simulink model "QuickStart"  (R2025a)
settings: Solver=VariableStepAuto  StartTime=0.0  StopTime=10.0  RelTol=1e-3
undefined symbols (not defined in the file): GND, GPIO, GPIO21, SCL, SDA
settings Model: Creator=el2jo  LastModifiedBy=el2jo

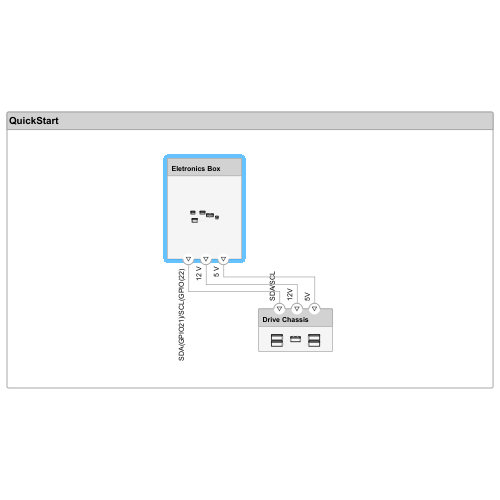
[thumbnail: Simulink's stored preview of the top-level diagram]
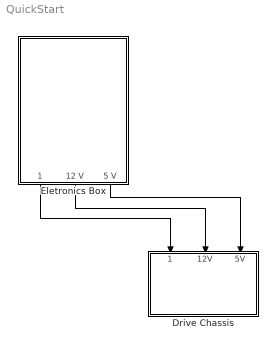
== system QuickStart ==
  Drive Chassis : Subsystem
      settings: PortSchema="{\"entries\":[{\"content\":{\"headerSize\":26,\"margin\":15,\"minimumSpacing\":25,\"sides\":[{\"content\":{},\"type\":\"ConnectorPlacement.EquallySpacedRectSide\",\"uuid\":\"48750758-9584-4908-8a58-a5fbbb9d9ec3\"},{\"content\":{\"side\":\"RIGHT\"},\"type\":\"ConnectorPlacement.EquallySpacedRectSide\",\"uuid\":\"52e2dad0-3097-421a-a882-362bd1258adc\"},{\"content\":{\"connectorIds\":[\"In1\",\"In2\",\"In3\"],\"side\":\"TOP\"},\"type\":\"ConnectorPlacement.EquallySpacedRectSide\",\"uuid\":\"e1803bf7-bd84-4e5d-8e9a-f8685f061664\"}]},\"type\":\"ConnectorPlacement.EquallySpacedConnector\",\"uuid\":\"5c436555-fc09-4a01-8a1e-11ce2b921fa0\"}],\"packageUris\":[\"http://schema.mathworks.com/mf0/Connector/R2020b\"],\"version\":\"1.0\"}"
  Eletronics Box : Subsystem
      settings: PortSchema="{\"entries\":[{\"content\":{\"headerSize\":26,\"margin\":15,\"minimumSpacing\":25,\"sides\":[{\"content\":{},\"type\":\"ConnectorPlacement.EquallySpacedRectSide\",\"uuid\":\"48750758-9584-4908-8a58-a5fbbb9d9ec3\"},{\"content\":{\"side\":\"RIGHT\"},\"type\":\"ConnectorPlacement.EquallySpacedRectSide\",\"uuid\":\"52e2dad0-3097-421a-a882-362bd1258adc\"},{\"content\":{\"side\":\"TOP\"},\"type\":\"ConnectorPlacement.EquallySpacedRectSide\",\"uuid\":\"e1803bf7-bd84-4e5d-8e9a-f8685f061664\"},{\"content\":{\"connectorIds\":[\"Out1\",\"Out2\",\"Out3\"],\"side\":\"BOTTOM\"},\"type\":\"ConnectorPlacement.EquallySpacedRectSide\",\"uuid\":\"9bfc03fe-8379-40b6-97ce-fe4ee1bc092f\"}]},\"type\":\"ConnectorPlacement.EquallySpacedConnector\",\"uuid\":\"5c436555-fc09-4a01-8a1e-11ce2b921fa0\"}],\"packageUris\":[\"http://schema.mathworks.com/mf0/Connector/R2020b\"],\"version\":\"1.0\"}"
  wires:
  Eletronics Box/3(5 V) -> Drive Chassis/3(5V)
  Eletronics Box/1("SDA(GPIO21)/SCL(GPIO(22) ") -> Drive Chassis/1(SDA/SCL)
  Eletronics Box/2(12 V) -> Drive Chassis/2(12V)

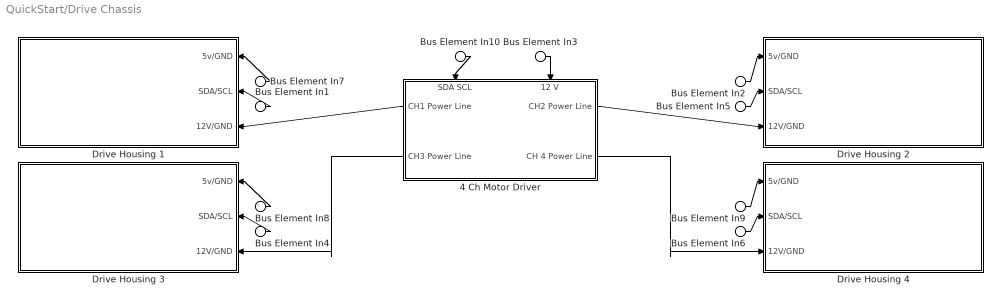
== system QuickStart/Drive Chassis ==
  Bus Element In{1,4..6,10} (5 alike) : Inport  PortName=SDA/SCL
  Bus Element In3 : Inport  Port=2  PortName=12V
  Bus Element In{2,7..9} (4 alike) : Inport  Port=3  PortName=5V
  4 Ch Motor Driver : Subsystem
      settings: PortSchema="{\"entries\":[{\"content\":{\"headerSize\":26,\"margin\":15,\"minimumSpacing\":25,\"sides\":[{\"content\":{\"connectorIds\":[\"Out1\",\"Out3\"]},\"type\":\"ConnectorPlacement.EquallySpacedRectSide\",\"uuid\":\"48750758-9584-4908-8a58-a5fbbb9d9ec3\"},{\"content\":{\"connectorIds\":[\"Out2\",\"Out4\"],\"side\":\"RIGHT\"},\"type\":\"ConnectorPlacement.EquallySpacedRectSide\",\"uuid\":\"52e2dad0-3097-421a-a882-362bd1258adc\"},{\"content\":{\"connectorIds\":[\"In1\",\"In2\"],\"side\":\"TOP\"},\"type\":\"ConnectorPlacement.EquallySpacedRectSide\",\"uuid\":\"e1803bf7-bd84-4e5d-8e9a-f8685f061664\"}]},\"type\":\"ConnectorPlacement.EquallySpacedConnector\",\"uuid\":\"5c436555-fc09-4a01-8a1e-11ce2b921fa0\"}],\"packageUris\":[\"http://schema.mathworks.com/mf0/Connector/R2020b\"],\"version\":\"1.0\"}"
  Drive Housing 1 : Subsystem
      settings: PortSchema="{\"entries\":[{\"content\":{\"headerSize\":26,\"margin\":15,\"minimumSpacing\":25,\"sides\":[{\"content\":{},\"type\":\"ConnectorPlacement.EquallySpacedRectSide\",\"uuid\":\"e7607396-8c96-4a6c-8f29-b5a2e3597902\"},{\"content\":{\"connectorIds\":[\"In1\",\"In2\",\"In3\"],\"side\":\"RIGHT\"},\"type\":\"ConnectorPlacement.EquallySpacedRectSide\",\"uuid\":\"459ece88-82a0-4a1d-ada4-6a68a35fe0a8\"},{\"content\":{\"side\":\"TOP\"},\"type\":\"ConnectorPlacement.EquallySpacedRectSide\",\"uuid\":\"796374a7-05ea-42d9-8bb3-fc90485df8c0\"}]},\"type\":\"ConnectorPlacement.EquallySpacedConnector\",\"uuid\":\"d0e626ee-7e22-4847-893e-8ab9090f2344\"}],\"packageUris\":[\"http://schema.mathworks.com/mf0/Connector/R2020b\"],\"version\":\"1.0\"}"
  Drive Housing 2 : Subsystem
      settings: PortSchema="{\"entries\":[{\"content\":{\"headerSize\":26,\"margin\":15,\"minimumSpacing\":25,\"sides\":[{\"content\":{\"connectorIds\":[\"In1\",\"In2\",\"In3\"]},\"type\":\"ConnectorPlacement.EquallySpacedRectSide\",\"uuid\":\"e7607396-8c96-4a6c-8f29-b5a2e3597902\"},{\"content\":{\"side\":\"RIGHT\"},\"type\":\"ConnectorPlacement.EquallySpacedRectSide\",\"uuid\":\"459ece88-82a0-4a1d-ada4-6a68a35fe0a8\"},{\"content\":{\"side\":\"TOP\"},\"type\":\"ConnectorPlacement.EquallySpacedRectSide\",\"uuid\":\"796374a7-05ea-42d9-8bb3-fc90485df8c0\"}]},\"type\":\"ConnectorPlacement.EquallySpacedConnector\",\"uuid\":\"d0e626ee-7e22-4847-893e-8ab9090f2344\"}],\"packageUris\":[\"http://schema.mathworks.com/mf0/Connector/R2020b\"],\"version\":\"1.0\"}"
  Drive Housing 3 : Subsystem
      settings: PortSchema="{\"entries\":[{\"content\":{\"headerSize\":26,\"margin\":15,\"minimumSpacing\":25,\"sides\":[{\"content\":{},\"type\":\"ConnectorPlacement.EquallySpacedRectSide\",\"uuid\":\"e7607396-8c96-4a6c-8f29-b5a2e3597902\"},{\"content\":{\"connectorIds\":[\"In1\",\"In2\",\"In3\"],\"side\":\"RIGHT\"},\"type\":\"ConnectorPlacement.EquallySpacedRectSide\",\"uuid\":\"459ece88-82a0-4a1d-ada4-6a68a35fe0a8\"},{\"content\":{\"side\":\"TOP\"},\"type\":\"ConnectorPlacement.EquallySpacedRectSide\",\"uuid\":\"796374a7-05ea-42d9-8bb3-fc90485df8c0\"}]},\"type\":\"ConnectorPlacement.EquallySpacedConnector\",\"uuid\":\"d0e626ee-7e22-4847-893e-8ab9090f2344\"}],\"packageUris\":[\"http://schema.mathworks.com/mf0/Connector/R2020b\"],\"version\":\"1.0\"}"
  Drive Housing 4 : Subsystem
      settings: PortSchema="{\"entries\":[{\"content\":{\"headerSize\":26,\"margin\":15,\"minimumSpacing\":25,\"sides\":[{\"content\":{\"connectorIds\":[\"In1\",\"In2\",\"In3\"]},\"type\":\"ConnectorPlacement.EquallySpacedRectSide\",\"uuid\":\"e7607396-8c96-4a6c-8f29-b5a2e3597902\"},{\"content\":{\"side\":\"RIGHT\"},\"type\":\"ConnectorPlacement.EquallySpacedRectSide\",\"uuid\":\"459ece88-82a0-4a1d-ada4-6a68a35fe0a8\"},{\"content\":{\"side\":\"TOP\"},\"type\":\"ConnectorPlacement.EquallySpacedRectSide\",\"uuid\":\"796374a7-05ea-42d9-8bb3-fc90485df8c0\"}]},\"type\":\"ConnectorPlacement.EquallySpacedConnector\",\"uuid\":\"d0e626ee-7e22-4847-893e-8ab9090f2344\"}],\"packageUris\":[\"http://schema.mathworks.com/mf0/Connector/R2020b\"],\"version\":\"1.0\"}"
  wires:
  4 Ch Motor Driver/4(CH 4 Power Line) -> Drive Housing 4/3(12V/GND)
  4 Ch Motor Driver/2(CH2 Power Line) -> Drive Housing 2/3(12V/GND)
  4 Ch Motor Driver/3(CH3 Power Line) -> Drive Housing 3/3(12V/GND)
  4 Ch Motor Driver/1(CH1 Power Line) -> Drive Housing 1/3(12V/GND)
  Bus Element In1/1 -> Drive Housing 1/2(SDA/SCL)
  Bus Element In4/1 -> Drive Housing 3/2(SDA/SCL)
  Bus Element In5/1 -> Drive Housing 2/2(SDA/SCL)
  Bus Element In6/1 -> Drive Housing 4/2(SDA/SCL)
  Bus Element In2/1 -> Drive Housing 2/1(5v/GND)
  Bus Element In7/1 -> Drive Housing 1/1(5v/GND)
  Bus Element In8/1 -> Drive Housing 3/1(5v/GND)
  Bus Element In9/1 -> Drive Housing 4/1(5v/GND)
  Bus Element In10/1 -> 4 Ch Motor Driver/1(SDA SCL)
  Bus Element In3/1 -> 4 Ch Motor Driver/2("12 V ")

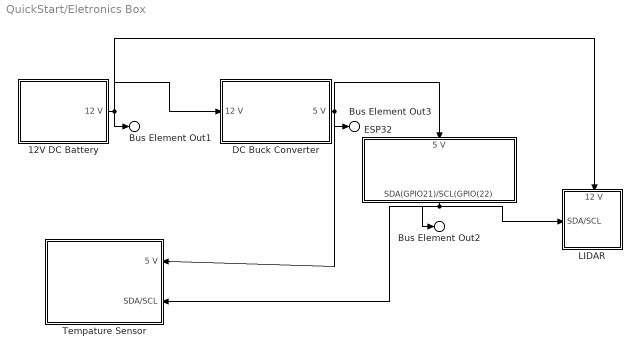
== system QuickStart/Eletronics Box ==
  12V DC Battery : Subsystem
      settings: PortSchema="{\"entries\":[{\"content\":{\"headerSize\":26,\"margin\":15,\"minimumSpacing\":25,\"sides\":[{\"content\":{},\"type\":\"ConnectorPlacement.EquallySpacedRectSide\",\"uuid\":\"48750758-9584-4908-8a58-a5fbbb9d9ec3\"},{\"content\":{\"connectorIds\":[\"Out1\"],\"side\":\"RIGHT\"},\"type\":\"ConnectorPlacement.EquallySpacedRectSide\",\"uuid\":\"52e2dad0-3097-421a-a882-362bd1258adc\"},{\"content\":{\"side\":\"TOP\"},\"type\":\"ConnectorPlacement.EquallySpacedRectSide\",\"uuid\":\"e1803bf7-bd84-4e5d-8e9a-f8685f061664\"}]},\"type\":\"ConnectorPlacement.EquallySpacedConnector\",\"uuid\":\"5c436555-fc09-4a01-8a1e-11ce2b921fa0\"}],\"packageUris\":[\"http://schema.mathworks.com/mf0/Connector/R2020b\"],\"version\":\"1.0\"}"
  DC Buck Converter : Subsystem
      settings: PortSchema="{\"entries\":[{\"content\":{\"headerSize\":26,\"margin\":15,\"minimumSpacing\":25,\"sides\":[{\"content\":{\"connectorIds\":[\"In1\"]},\"type\":\"ConnectorPlacement.EquallySpacedRectSide\",\"uuid\":\"48750758-9584-4908-8a58-a5fbbb9d9ec3\"},{\"content\":{\"connectorIds\":[\"Out1\"],\"side\":\"RIGHT\"},\"type\":\"ConnectorPlacement.EquallySpacedRectSide\",\"uuid\":\"52e2dad0-3097-421a-a882-362bd1258adc\"},{\"content\":{\"side\":\"TOP\"},\"type\":\"ConnectorPlacement.EquallySpacedRectSide\",\"uuid\":\"e1803bf7-bd84-4e5d-8e9a-f8685f061664\"}]},\"type\":\"ConnectorPlacement.EquallySpacedConnector\",\"uuid\":\"5c436555-fc09-4a01-8a1e-11ce2b921fa0\"}],\"packageUris\":[\"http://schema.mathworks.com/mf0/Connector/R2020b\"],\"version\":\"1.0\"}"
  ESP32 : Subsystem
      settings: PortSchema="{\"entries\":[{\"content\":{\"headerSize\":26,\"margin\":15,\"minimumSpacing\":25,\"sides\":[{\"content\":{},\"type\":\"ConnectorPlacement.EquallySpacedRectSide\",\"uuid\":\"48750758-9584-4908-8a58-a5fbbb9d9ec3\"},{\"content\":{\"side\":\"RIGHT\"},\"type\":\"ConnectorPlacement.EquallySpacedRectSide\",\"uuid\":\"52e2dad0-3097-421a-a882-362bd1258adc\"},{\"content\":{\"connectorIds\":[\"In1\"],\"side\":\"TOP\"},\"type\":\"ConnectorPlacement.EquallySpacedRectSide\",\"uuid\":\"e1803bf7-bd84-4e5d-8e9a-f8685f061664\"},{\"content\":{\"connectorIds\":[\"Out1\"],\"side\":\"BOTTOM\"},\"type\":\"ConnectorPlacement.EquallySpacedRectSide\",\"uuid\":\"3c1c43d4-aa76-4122-9080-ecb1da993d45\"}]},\"type\":\"ConnectorPlacement.EquallySpacedConnector\",\"uuid\":\"5c436555-fc09-4a01-8a1e-11ce2b921fa0\"}],\"packageUris\":[\"http://schema.mathworks.com/mf0/Connector/R2020b\"],\"version\":\"1.0\"}"
  LIDAR : Subsystem
      settings: PortSchema="{\"entries\":[{\"content\":{\"headerSize\":26,\"margin\":15,\"minimumSpacing\":25,\"sides\":[{\"content\":{\"connectorIds\":[\"In1\"]},\"type\":\"ConnectorPlacement.EquallySpacedRectSide\",\"uuid\":\"48750758-9584-4908-8a58-a5fbbb9d9ec3\"},{\"content\":{\"side\":\"RIGHT\"},\"type\":\"ConnectorPlacement.EquallySpacedRectSide\",\"uuid\":\"52e2dad0-3097-421a-a882-362bd1258adc\"},{\"content\":{\"connectorIds\":[\"In2\"],\"side\":\"TOP\"},\"type\":\"ConnectorPlacement.EquallySpacedRectSide\",\"uuid\":\"e1803bf7-bd84-4e5d-8e9a-f8685f061664\"}]},\"type\":\"ConnectorPlacement.EquallySpacedConnector\",\"uuid\":\"5c436555-fc09-4a01-8a1e-11ce2b921fa0\"}],\"packageUris\":[\"http://schema.mathworks.com/mf0/Connector/R2020b\"],\"version\":\"1.0\"}"
  Tempature Sensor : Subsystem
      settings: PortSchema="{\"entries\":[{\"content\":{\"headerSize\":26,\"margin\":15,\"minimumSpacing\":25,\"sides\":[{\"content\":{},\"type\":\"ConnectorPlacement.EquallySpacedRectSide\",\"uuid\":\"48750758-9584-4908-8a58-a5fbbb9d9ec3\"},{\"content\":{\"connectorIds\":[\"In1\",\"In2\"],\"side\":\"RIGHT\"},\"type\":\"ConnectorPlacement.EquallySpacedRectSide\",\"uuid\":\"52e2dad0-3097-421a-a882-362bd1258adc\"},{\"content\":{\"side\":\"TOP\"},\"type\":\"ConnectorPlacement.EquallySpacedRectSide\",\"uuid\":\"e1803bf7-bd84-4e5d-8e9a-f8685f061664\"}]},\"type\":\"ConnectorPlacement.EquallySpacedConnector\",\"uuid\":\"5c436555-fc09-4a01-8a1e-11ce2b921fa0\"}],\"packageUris\":[\"http://schema.mathworks.com/mf0/Connector/R2020b\"],\"version\":\"1.0\"}"
  Bus Element Out2 : Outport  PortName=SDA(GPIO21)/SCL(GPIO(22)
  Bus Element Out1 : Outport  Port=2  PortName=12 V
  Bus Element Out3 : Outport  Port=3  PortName=5 V
  wires:
  12V DC Battery/1(12 V) -> Bus Element Out1/1, DC Buck Converter/1(12 V), LIDAR/2(12 V)
  ESP32/1("SDA(GPIO21)/SCL(GPIO(22) ") -> Bus Element Out2/1, Tempature Sensor/2(SDA/SCL), LIDAR/1(SDA/SCL)
  DC Buck Converter/1(5 V) -> Bus Element Out3/1, Tempature Sensor/1(5 V), ESP32/1(5 V)

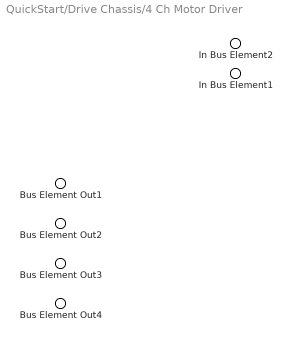
== system QuickStart/Drive Chassis/4 Ch Motor Driver ==
  In Bus Element1 : Inport  PortName=SDA SCL
  In Bus Element2 : Inport  Port=2  PortName=12 V
  Bus Element Out1 : Outport  PortName=CH1 Power Line
  Bus Element Out2 : Outport  Port=2  PortName=CH2 Power Line
  Bus Element Out3 : Outport  Port=3  PortName=CH3 Power Line
  Bus Element Out4 : Outport  Port=4  PortName=CH 4 Power Line

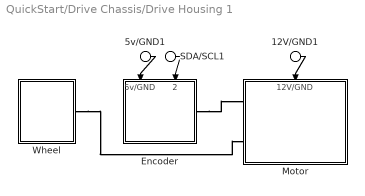
== system QuickStart/Drive Chassis/Drive Housing 1 ==
  5v/GND1 : Inport  PortName=5v/GND
  SDA/SCL1 : Inport  Port=2  PortName=SDA/SCL
  12V/GND1 : Inport  Port=3  PortName=12V/GND
  "Encoder " : Subsystem
      settings: PortSchema="{\"entries\":[{\"content\":{\"headerSize\":26,\"margin\":15,\"minimumSpacing\":25,\"sides\":[{\"content\":{},\"type\":\"ConnectorPlacement.EquallySpacedRectSide\",\"uuid\":\"48750758-9584-4908-8a58-a5fbbb9d9ec3\"},{\"content\":{\"connectorIds\":[\"RConn1\"],\"side\":\"RIGHT\"},\"type\":\"ConnectorPlacement.EquallySpacedRectSide\",\"uuid\":\"52e2dad0-3097-421a-a882-362bd1258adc\"},{\"content\":{\"connectorIds\":[\"In1\",\"In2\"],\"side\":\"TOP\"},\"type\":\"ConnectorPlacement.EquallySpacedRectSide\",\"uuid\":\"e1803bf7-bd84-4e5d-8e9a-f8685f061664\"}]},\"type\":\"ConnectorPlacement.EquallySpacedConnector\",\"uuid\":\"5c436555-fc09-4a01-8a1e-11ce2b921fa0\"}],\"packageUris\":[\"http://schema.mathworks.com/mf0/Connector/R2020b\"],\"version\":\"1.0\"}"
  Motor : Subsystem
      settings: PortSchema="{\"entries\":[{\"content\":{\"headerSize\":26,\"margin\":15,\"minimumSpacing\":25,\"sides\":[{\"content\":{\"connectorIds\":[\"LConn1\",\"LConn2\"]},\"type\":\"ConnectorPlacement.EquallySpacedRectSide\",\"uuid\":\"48750758-9584-4908-8a58-a5fbbb9d9ec3\"},{\"content\":{\"side\":\"RIGHT\"},\"type\":\"ConnectorPlacement.EquallySpacedRectSide\",\"uuid\":\"52e2dad0-3097-421a-a882-362bd1258adc\"},{\"content\":{\"connectorIds\":[\"In1\"],\"side\":\"TOP\"},\"type\":\"ConnectorPlacement.EquallySpacedRectSide\",\"uuid\":\"e1803bf7-bd84-4e5d-8e9a-f8685f061664\"}]},\"type\":\"ConnectorPlacement.EquallySpacedConnector\",\"uuid\":\"5c436555-fc09-4a01-8a1e-11ce2b921fa0\"}],\"packageUris\":[\"http://schema.mathworks.com/mf0/Connector/R2020b\"],\"version\":\"1.0\"}"
  Wheel : Subsystem
      settings: PortSchema="{\"entries\":[{\"content\":{\"headerSize\":26,\"margin\":15,\"minimumSpacing\":25,\"sides\":[{\"content\":{},\"type\":\"ConnectorPlacement.EquallySpacedRectSide\",\"uuid\":\"48750758-9584-4908-8a58-a5fbbb9d9ec3\"},{\"content\":{\"connectorIds\":[\"RConn1\"],\"side\":\"RIGHT\"},\"type\":\"ConnectorPlacement.EquallySpacedRectSide\",\"uuid\":\"52e2dad0-3097-421a-a882-362bd1258adc\"},{\"content\":{\"side\":\"TOP\"},\"type\":\"ConnectorPlacement.EquallySpacedRectSide\",\"uuid\":\"e1803bf7-bd84-4e5d-8e9a-f8685f061664\"}]},\"type\":\"ConnectorPlacement.EquallySpacedConnector\",\"uuid\":\"5c436555-fc09-4a01-8a1e-11ce2b921fa0\"}],\"packageUris\":[\"http://schema.mathworks.com/mf0/Connector/R2020b\"],\"version\":\"1.0\"}"
  wires:
  5v/GND1/1 -> "Encoder "/1(5v/GND)
  SDA/SCL1/1 -> "Encoder "/2(SDA/SCL)
  12V/GND1/1 -> Motor/1(12V/GND)
  connections:
  "Encoder "/RConn1 -- Motor/LConn1
  Wheel/RConn1 -- Motor/LConn2

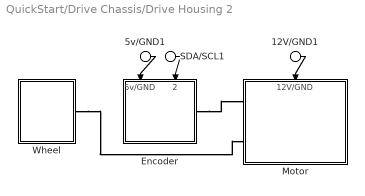
== system QuickStart/Drive Chassis/Drive Housing 2 ==
  5v/GND1 : Inport  PortName=5v/GND
  SDA/SCL1 : Inport  Port=2  PortName=SDA/SCL
  12V/GND1 : Inport  Port=3  PortName=12V/GND
  "Encoder " : Subsystem
      settings: PortSchema="{\"entries\":[{\"content\":{\"headerSize\":26,\"margin\":15,\"minimumSpacing\":25,\"sides\":[{\"content\":{},\"type\":\"ConnectorPlacement.EquallySpacedRectSide\",\"uuid\":\"48750758-9584-4908-8a58-a5fbbb9d9ec3\"},{\"content\":{\"connectorIds\":[\"RConn1\"],\"side\":\"RIGHT\"},\"type\":\"ConnectorPlacement.EquallySpacedRectSide\",\"uuid\":\"52e2dad0-3097-421a-a882-362bd1258adc\"},{\"content\":{\"connectorIds\":[\"In1\",\"In2\"],\"side\":\"TOP\"},\"type\":\"ConnectorPlacement.EquallySpacedRectSide\",\"uuid\":\"e1803bf7-bd84-4e5d-8e9a-f8685f061664\"}]},\"type\":\"ConnectorPlacement.EquallySpacedConnector\",\"uuid\":\"5c436555-fc09-4a01-8a1e-11ce2b921fa0\"}],\"packageUris\":[\"http://schema.mathworks.com/mf0/Connector/R2020b\"],\"version\":\"1.0\"}"
  Motor : Subsystem
      settings: PortSchema="{\"entries\":[{\"content\":{\"headerSize\":26,\"margin\":15,\"minimumSpacing\":25,\"sides\":[{\"content\":{\"connectorIds\":[\"LConn1\",\"LConn2\"]},\"type\":\"ConnectorPlacement.EquallySpacedRectSide\",\"uuid\":\"48750758-9584-4908-8a58-a5fbbb9d9ec3\"},{\"content\":{\"side\":\"RIGHT\"},\"type\":\"ConnectorPlacement.EquallySpacedRectSide\",\"uuid\":\"52e2dad0-3097-421a-a882-362bd1258adc\"},{\"content\":{\"connectorIds\":[\"In1\"],\"side\":\"TOP\"},\"type\":\"ConnectorPlacement.EquallySpacedRectSide\",\"uuid\":\"e1803bf7-bd84-4e5d-8e9a-f8685f061664\"}]},\"type\":\"ConnectorPlacement.EquallySpacedConnector\",\"uuid\":\"5c436555-fc09-4a01-8a1e-11ce2b921fa0\"}],\"packageUris\":[\"http://schema.mathworks.com/mf0/Connector/R2020b\"],\"version\":\"1.0\"}"
  Wheel : Subsystem
      settings: PortSchema="{\"entries\":[{\"content\":{\"headerSize\":26,\"margin\":15,\"minimumSpacing\":25,\"sides\":[{\"content\":{},\"type\":\"ConnectorPlacement.EquallySpacedRectSide\",\"uuid\":\"48750758-9584-4908-8a58-a5fbbb9d9ec3\"},{\"content\":{\"connectorIds\":[\"RConn1\"],\"side\":\"RIGHT\"},\"type\":\"ConnectorPlacement.EquallySpacedRectSide\",\"uuid\":\"52e2dad0-3097-421a-a882-362bd1258adc\"},{\"content\":{\"side\":\"TOP\"},\"type\":\"ConnectorPlacement.EquallySpacedRectSide\",\"uuid\":\"e1803bf7-bd84-4e5d-8e9a-f8685f061664\"}]},\"type\":\"ConnectorPlacement.EquallySpacedConnector\",\"uuid\":\"5c436555-fc09-4a01-8a1e-11ce2b921fa0\"}],\"packageUris\":[\"http://schema.mathworks.com/mf0/Connector/R2020b\"],\"version\":\"1.0\"}"
  wires:
  5v/GND1/1 -> "Encoder "/1(5v/GND)
  SDA/SCL1/1 -> "Encoder "/2(SDA/SCL)
  12V/GND1/1 -> Motor/1(12V/GND)
  connections:
  "Encoder "/RConn1 -- Motor/LConn1
  Wheel/RConn1 -- Motor/LConn2

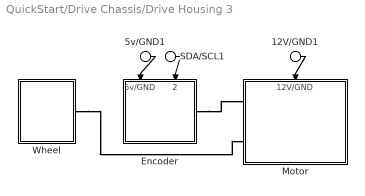
== system QuickStart/Drive Chassis/Drive Housing 3 ==
  5v/GND1 : Inport  PortName=5v/GND
  SDA/SCL1 : Inport  Port=2  PortName=SDA/SCL
  12V/GND1 : Inport  Port=3  PortName=12V/GND
  "Encoder " : Subsystem
      settings: PortSchema="{\"entries\":[{\"content\":{\"headerSize\":26,\"margin\":15,\"minimumSpacing\":25,\"sides\":[{\"content\":{},\"type\":\"ConnectorPlacement.EquallySpacedRectSide\",\"uuid\":\"48750758-9584-4908-8a58-a5fbbb9d9ec3\"},{\"content\":{\"connectorIds\":[\"RConn1\"],\"side\":\"RIGHT\"},\"type\":\"ConnectorPlacement.EquallySpacedRectSide\",\"uuid\":\"52e2dad0-3097-421a-a882-362bd1258adc\"},{\"content\":{\"connectorIds\":[\"In1\",\"In2\"],\"side\":\"TOP\"},\"type\":\"ConnectorPlacement.EquallySpacedRectSide\",\"uuid\":\"e1803bf7-bd84-4e5d-8e9a-f8685f061664\"}]},\"type\":\"ConnectorPlacement.EquallySpacedConnector\",\"uuid\":\"5c436555-fc09-4a01-8a1e-11ce2b921fa0\"}],\"packageUris\":[\"http://schema.mathworks.com/mf0/Connector/R2020b\"],\"version\":\"1.0\"}"
  Motor : Subsystem
      settings: PortSchema="{\"entries\":[{\"content\":{\"headerSize\":26,\"margin\":15,\"minimumSpacing\":25,\"sides\":[{\"content\":{\"connectorIds\":[\"LConn1\",\"LConn2\"]},\"type\":\"ConnectorPlacement.EquallySpacedRectSide\",\"uuid\":\"48750758-9584-4908-8a58-a5fbbb9d9ec3\"},{\"content\":{\"side\":\"RIGHT\"},\"type\":\"ConnectorPlacement.EquallySpacedRectSide\",\"uuid\":\"52e2dad0-3097-421a-a882-362bd1258adc\"},{\"content\":{\"connectorIds\":[\"In1\"],\"side\":\"TOP\"},\"type\":\"ConnectorPlacement.EquallySpacedRectSide\",\"uuid\":\"e1803bf7-bd84-4e5d-8e9a-f8685f061664\"}]},\"type\":\"ConnectorPlacement.EquallySpacedConnector\",\"uuid\":\"5c436555-fc09-4a01-8a1e-11ce2b921fa0\"}],\"packageUris\":[\"http://schema.mathworks.com/mf0/Connector/R2020b\"],\"version\":\"1.0\"}"
  Wheel : Subsystem
      settings: PortSchema="{\"entries\":[{\"content\":{\"headerSize\":26,\"margin\":15,\"minimumSpacing\":25,\"sides\":[{\"content\":{},\"type\":\"ConnectorPlacement.EquallySpacedRectSide\",\"uuid\":\"48750758-9584-4908-8a58-a5fbbb9d9ec3\"},{\"content\":{\"connectorIds\":[\"RConn1\"],\"side\":\"RIGHT\"},\"type\":\"ConnectorPlacement.EquallySpacedRectSide\",\"uuid\":\"52e2dad0-3097-421a-a882-362bd1258adc\"},{\"content\":{\"side\":\"TOP\"},\"type\":\"ConnectorPlacement.EquallySpacedRectSide\",\"uuid\":\"e1803bf7-bd84-4e5d-8e9a-f8685f061664\"}]},\"type\":\"ConnectorPlacement.EquallySpacedConnector\",\"uuid\":\"5c436555-fc09-4a01-8a1e-11ce2b921fa0\"}],\"packageUris\":[\"http://schema.mathworks.com/mf0/Connector/R2020b\"],\"version\":\"1.0\"}"
  wires:
  5v/GND1/1 -> "Encoder "/1(5v/GND)
  SDA/SCL1/1 -> "Encoder "/2(SDA/SCL)
  12V/GND1/1 -> Motor/1(12V/GND)
  connections:
  "Encoder "/RConn1 -- Motor/LConn1
  Wheel/RConn1 -- Motor/LConn2

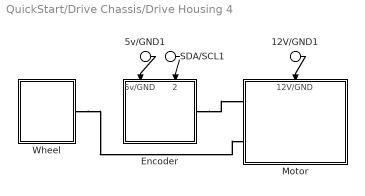
== system QuickStart/Drive Chassis/Drive Housing 4 ==
  5v/GND1 : Inport  PortName=5v/GND
  SDA/SCL1 : Inport  Port=2  PortName=SDA/SCL
  12V/GND1 : Inport  Port=3  PortName=12V/GND
  "Encoder " : Subsystem
      settings: PortSchema="{\"entries\":[{\"content\":{\"headerSize\":26,\"margin\":15,\"minimumSpacing\":25,\"sides\":[{\"content\":{},\"type\":\"ConnectorPlacement.EquallySpacedRectSide\",\"uuid\":\"48750758-9584-4908-8a58-a5fbbb9d9ec3\"},{\"content\":{\"connectorIds\":[\"RConn1\"],\"side\":\"RIGHT\"},\"type\":\"ConnectorPlacement.EquallySpacedRectSide\",\"uuid\":\"52e2dad0-3097-421a-a882-362bd1258adc\"},{\"content\":{\"connectorIds\":[\"In1\",\"In2\"],\"side\":\"TOP\"},\"type\":\"ConnectorPlacement.EquallySpacedRectSide\",\"uuid\":\"e1803bf7-bd84-4e5d-8e9a-f8685f061664\"}]},\"type\":\"ConnectorPlacement.EquallySpacedConnector\",\"uuid\":\"5c436555-fc09-4a01-8a1e-11ce2b921fa0\"}],\"packageUris\":[\"http://schema.mathworks.com/mf0/Connector/R2020b\"],\"version\":\"1.0\"}"
  Motor : Subsystem
      settings: PortSchema="{\"entries\":[{\"content\":{\"headerSize\":26,\"margin\":15,\"minimumSpacing\":25,\"sides\":[{\"content\":{\"connectorIds\":[\"LConn1\",\"LConn2\"]},\"type\":\"ConnectorPlacement.EquallySpacedRectSide\",\"uuid\":\"48750758-9584-4908-8a58-a5fbbb9d9ec3\"},{\"content\":{\"side\":\"RIGHT\"},\"type\":\"ConnectorPlacement.EquallySpacedRectSide\",\"uuid\":\"52e2dad0-3097-421a-a882-362bd1258adc\"},{\"content\":{\"connectorIds\":[\"In1\"],\"side\":\"TOP\"},\"type\":\"ConnectorPlacement.EquallySpacedRectSide\",\"uuid\":\"e1803bf7-bd84-4e5d-8e9a-f8685f061664\"}]},\"type\":\"ConnectorPlacement.EquallySpacedConnector\",\"uuid\":\"5c436555-fc09-4a01-8a1e-11ce2b921fa0\"}],\"packageUris\":[\"http://schema.mathworks.com/mf0/Connector/R2020b\"],\"version\":\"1.0\"}"
  Wheel : Subsystem
      settings: PortSchema="{\"entries\":[{\"content\":{\"headerSize\":26,\"margin\":15,\"minimumSpacing\":25,\"sides\":[{\"content\":{},\"type\":\"ConnectorPlacement.EquallySpacedRectSide\",\"uuid\":\"48750758-9584-4908-8a58-a5fbbb9d9ec3\"},{\"content\":{\"connectorIds\":[\"RConn1\"],\"side\":\"RIGHT\"},\"type\":\"ConnectorPlacement.EquallySpacedRectSide\",\"uuid\":\"52e2dad0-3097-421a-a882-362bd1258adc\"},{\"content\":{\"side\":\"TOP\"},\"type\":\"ConnectorPlacement.EquallySpacedRectSide\",\"uuid\":\"e1803bf7-bd84-4e5d-8e9a-f8685f061664\"}]},\"type\":\"ConnectorPlacement.EquallySpacedConnector\",\"uuid\":\"5c436555-fc09-4a01-8a1e-11ce2b921fa0\"}],\"packageUris\":[\"http://schema.mathworks.com/mf0/Connector/R2020b\"],\"version\":\"1.0\"}"
  wires:
  5v/GND1/1 -> "Encoder "/1(5v/GND)
  SDA/SCL1/1 -> "Encoder "/2(SDA/SCL)
  12V/GND1/1 -> Motor/1(12V/GND)
  connections:
  "Encoder "/RConn1 -- Motor/LConn1
  Wheel/RConn1 -- Motor/LConn2

== system QuickStart/Eletronics Box/12V DC Battery ==
  Bus Element Out1 : Outport  PortName=12 V

== system QuickStart/Eletronics Box/DC Buck Converter ==
  Bus Element In1 : Inport  PortName=12 V
  Bus Element Out1 : Outport  PortName=5 V

== system QuickStart/Eletronics Box/ESP32 ==
  Bus Element In1 : Inport  PortName=5 V
  Bus Element Out1 : Outport  PortName=SDA(GPIO21)/SCL(GPIO(22)

== system QuickStart/Eletronics Box/LIDAR ==
  Bus Element In2 : Inport  PortName=SDA/SCL
  Bus Element In1 : Inport  Port=2  PortName=12 V

== system QuickStart/Eletronics Box/Tempature Sensor ==
  Bus Element In2 : Inport  PortName=5 V
  Bus Element In1 : Inport  Port=2  PortName=SDA/SCL

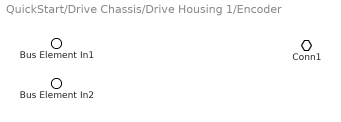
== system QuickStart/Drive Chassis/Drive Housing 1/Encoder  ==
  Bus Element In1 : Inport  PortName=5v/GND
  Bus Element In2 : Inport  Port=2  PortName=SDA/SCL
  Conn1 : PMIOPort  Side=Right

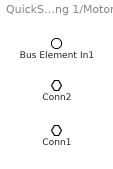
== system QuickStart/Drive Chassis/Drive Housing 1/Motor ==
  Bus Element In1 : Inport  PortName=12V/GND
  Conn2 : PMIOPort  Side=Left
  Conn1 : PMIOPort  Port=2  Side=Left

== system QuickStart/Drive Chassis/Drive Housing 1/Wheel ==
  Conn1 : PMIOPort  Side=Right

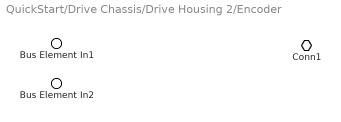
== system QuickStart/Drive Chassis/Drive Housing 2/Encoder  ==
  Bus Element In1 : Inport  PortName=5v/GND
  Bus Element In2 : Inport  Port=2  PortName=SDA/SCL
  Conn1 : PMIOPort  Side=Right

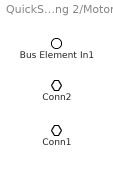
== system QuickStart/Drive Chassis/Drive Housing 2/Motor ==
  Bus Element In1 : Inport  PortName=12V/GND
  Conn2 : PMIOPort  Side=Left
  Conn1 : PMIOPort  Port=2  Side=Left

== system QuickStart/Drive Chassis/Drive Housing 2/Wheel ==
  Conn1 : PMIOPort  Side=Right

== system QuickStart/Drive Chassis/Drive Housing 3/Encoder  ==
  Bus Element In1 : Inport  PortName=5v/GND
  Bus Element In2 : Inport  Port=2  PortName=SDA/SCL
  Conn1 : PMIOPort  Side=Right

== system QuickStart/Drive Chassis/Drive Housing 3/Motor ==
  Bus Element In1 : Inport  PortName=12V/GND
  Conn2 : PMIOPort  Side=Left
  Conn1 : PMIOPort  Port=2  Side=Left

== system QuickStart/Drive Chassis/Drive Housing 3/Wheel ==
  Conn1 : PMIOPort  Side=Right

== system QuickStart/Drive Chassis/Drive Housing 4/Encoder  ==
  Bus Element In1 : Inport  PortName=5v/GND
  Bus Element In2 : Inport  Port=2  PortName=SDA/SCL
  Conn1 : PMIOPort  Side=Right

== system QuickStart/Drive Chassis/Drive Housing 4/Motor ==
  Bus Element In1 : Inport  PortName=12V/GND
  Conn2 : PMIOPort  Side=Left
  Conn1 : PMIOPort  Port=2  Side=Left

== system QuickStart/Drive Chassis/Drive Housing 4/Wheel ==
  Conn1 : PMIOPort  Side=Right
